simulink model "ProcessNetworkSimulation"  (R2018b)
settings: Solver=VariableStepAuto  StartTime=0.0  StopTime=2000  RelTol=1e-3  EnableMultiTasking=on
libraries: simulink x1, simeventslib x1
settings Model: Creator=tsprock3  LastModifiedBy=tas5
settings DataIOCC: LimitDataPoints=on
settings OptimizationCC: LifeSpan=inf
settings DebuggingCC: AllowSymbolicDim=off  SFUnexpectedBacktrackingDiag=warning  SFNoUnconditionalDefaultTransitionDiag=warning  SFExecutionAtInitializationDiag=none
settings ModelReferenceCC: PropagateSignalLabelsOutOfModel=off
settings SFSimCC: SimUseLocalCustomCode=off
settings RTWCC: RTWUseLocalCustomCode=off
settings CodeAppCC: StateflowObjectComments=on
settings GRTTargetCC: TargetLangStandard=C89/C90 (ANSI)
settings ConfigComp: CovMetricSettings=dw  CovHtmlReporting=on  CovSaveCumulativeToWorkspaceVar=on  CovSaveSingleToWorkspaceVar=on  CovExternalEMLEnable=off

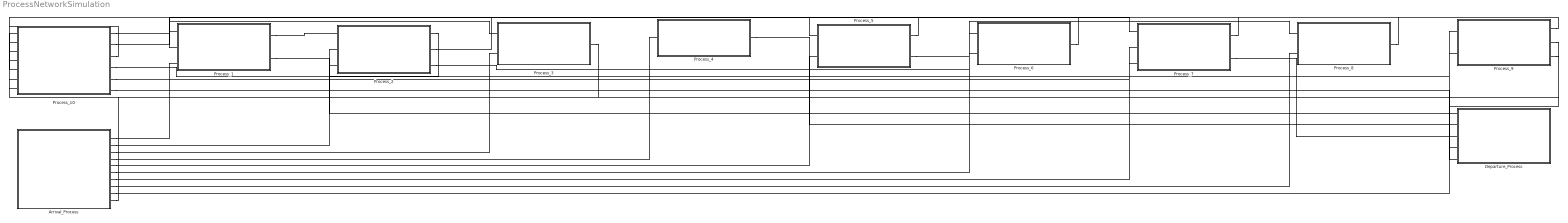
== system ProcessNetworkSimulation ==
  Arrival_Process : Subsystem
  Departure_Process : Subsystem
  Process_1 : Subsystem
  Process_10 : Subsystem
  Process_2 : Subsystem
  Process_3 : Subsystem
  Process_4 : Subsystem
  Process_5 : Subsystem
  Process_6 : Subsystem
  Process_7 : Subsystem
  Process_8 : Subsystem
  Process_9 : Subsystem
  connections:
  Process_9/RConn1 -- Process_1/LConn1
  Process_1/RConn1 -- Process_2/LConn1
  Process_2/RConn1 -- Process_2/LConn2
  Process_2/RConn2 -- Process_7/LConn1
  Process_10/RConn1 -- Process_3/LConn1
  Process_3/RConn1 -- Process_10/LConn1
  Process_10/RConn2 -- Process_5/LConn1
  Process_5/RConn1 -- Process_1/LConn2
  Process_2/RConn3 -- Process_6/LConn1
  Process_6/RConn1 -- Process_10/LConn2
  Process_10/RConn3 -- Process_10/LConn3
  Process_10/RConn4 -- Process_9/LConn1
  Process_5/RConn2 -- Process_8/LConn1
  Process_8/RConn1 -- Process_10/LConn4
  Process_7/RConn1 -- Process_10/LConn5
  Process_9/RConn2 -- Process_10/LConn6
  Process_10/RConn5 -- Process_7/LConn2
  Arrival_Process/RConn1 -- Process_1/LConn3
  Arrival_Process/RConn2 -- Process_2/LConn3
  Arrival_Process/RConn3 -- Process_3/LConn2
  Arrival_Process/RConn4 -- Process_4/LConn1
  Arrival_Process/RConn5 -- Process_5/LConn2
  Arrival_Process/RConn6 -- Process_6/LConn2
  Arrival_Process/RConn7 -- Process_7/LConn3
  Arrival_Process/RConn8 -- Process_8/LConn2
  Arrival_Process/RConn9 -- Process_9/LConn2
  Arrival_Process/RConn10 -- Process_10/LConn7
  Process_1/RConn2 -- Departure_Process/LConn1
  Process_4/RConn1 -- Departure_Process/LConn2
  Process_7/RConn2 -- Departure_Process/LConn3
  Process_9/RConn3 -- Departure_Process/LConn4
  Process_10/RConn6 -- Departure_Process/LConn5

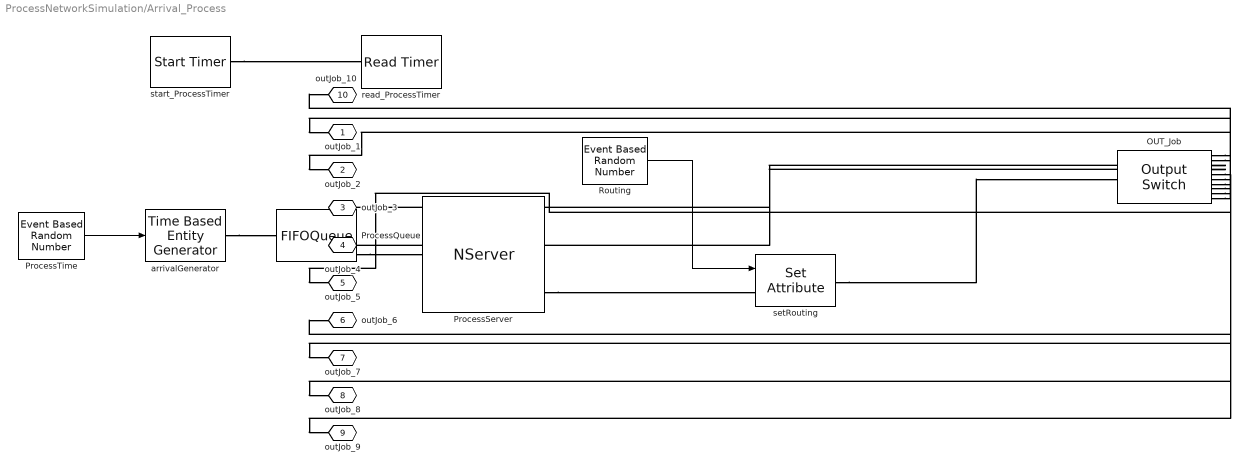
== system ProcessNetworkSimulation/Arrival_Process ==
  OUT_Job : OutputSwitch  NumberOutputPorts=10  SwitchingCriterion=From attribute  AttributeName=outputFlowNode
  ProcessQueue : FIFOQueue  Capacity=Inf  StatAverageWait=on  StatAverageQueueLength=on
      settings: OutputPortMap=o2,o3
  ProcessServer : NServer  NumberOfServers=Inf  ServiceTime=0  StatNumberDeparted=on  StatUtilization=on
      settings: OutputPortMap=o0,o5
  ProcessTime : EventBasedRandomNumber  meanExp=0.034483  minUnif=1  meanNorm=2  stdNorm=0.2  Seed=65399
  Routing : EventBasedRandomNumber  Distribution=Arbitrary discrete  valueVecDisc=[0,1,2,3,4,5,6,7,8,9,10]  probVecDisc=[0,0,0.1379,0,0,0,0,0.069,0,0.2759,0.5172]  Seed=3080
  arrivalGenerator : TimeBasedEntityGenerator  GenerateEntitiesUpon=Intergeneration time from port t
  read_ProcessTimer : ReadTimer  TimerTag=T_Arrival_Process  StatAverageTimeElapsed=on
      settings: OutputPortMap=o3
  setRouting : SetAttribute  AttributeName=outputFlowNode  AttributeFrom=Signal port  EvaluatedAttributeValue={ []}
  start_ProcessTimer : StartTimer  TimerTag=T_Arrival_Process  TimerStartedOption=Restart
  outJob_1 : PMIOPort  Side=Right
  outJob_2 : PMIOPort  Port=2  Side=Right
  outJob_3 : PMIOPort  Port=3  Side=Right
  outJob_4 : PMIOPort  Port=4  Side=Right
  outJob_5 : PMIOPort  Port=5  Side=Right
  outJob_6 : PMIOPort  Port=6  Side=Right
  outJob_7 : PMIOPort  Port=7  Side=Right
  outJob_8 : PMIOPort  Port=8  Side=Right
  outJob_9 : PMIOPort  Port=9  Side=Right
  outJob_10 : PMIOPort  Port=10  Side=Right
  wires:
  ProcessTime/1 -> arrivalGenerator/1
  Routing/1 -> setRouting/1
  connections:
  ProcessQueue/RConn1 -- ProcessServer/LConn1
  start_ProcessTimer/RConn1 -- read_ProcessTimer/LConn1
  arrivalGenerator/RConn1 -- ProcessQueue/LConn1
  ProcessServer/RConn1 -- setRouting/LConn1
  setRouting/RConn1 -- OUT_Job/LConn1
  OUT_Job/RConn1 -- outJob_1/RConn1
  OUT_Job/RConn2 -- outJob_2/RConn1
  OUT_Job/RConn3 -- outJob_3/RConn1
  OUT_Job/RConn4 -- outJob_4/RConn1
  OUT_Job/RConn5 -- outJob_5/RConn1
  OUT_Job/RConn6 -- outJob_6/RConn1
  OUT_Job/RConn7 -- outJob_7/RConn1
  OUT_Job/RConn8 -- outJob_8/RConn1
  OUT_Job/RConn9 -- outJob_9/RConn1
  OUT_Job/RConn10 -- outJob_10/RConn1

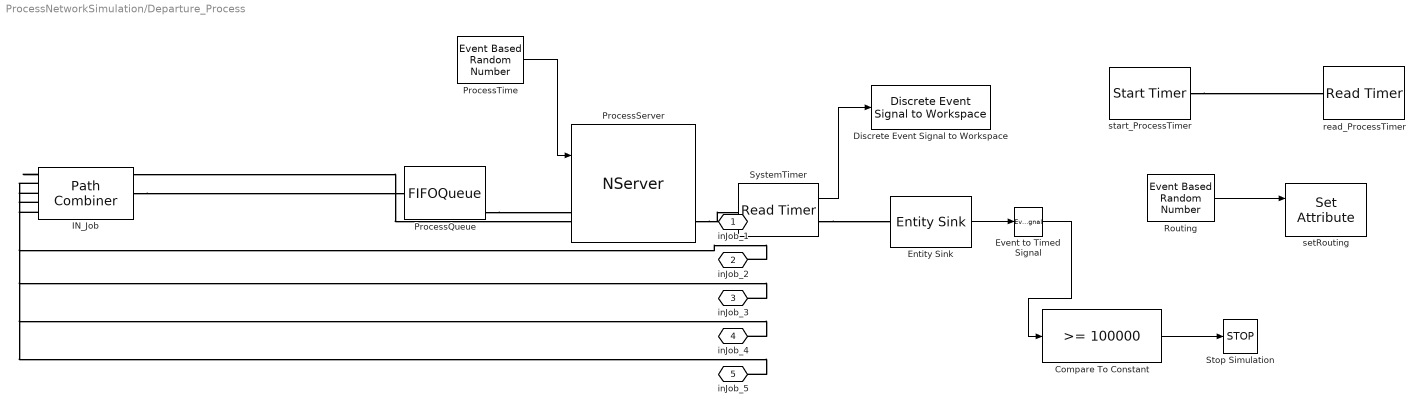
== system ProcessNetworkSimulation/Departure_Process ==
  Compare To Constant : simulink/Logic and Bit Operations/Compare To Constant  relop=>=  const=100000  OutDataTypeStr=boolean
  Discrete Event Signal to Workspace : simeventslib/SimEvents Sinks/Discrete Event Signal to Workspace  VariableName=ProcessTime  SaveFormat=Structure With Time  isMonitorOnly=off  isRecordIC=off
      settings: SourceProductName=SimEvents  SourceProductBaseCode=SE
  Entity Sink : EntitySink  StatNumberArrived=on
  Event to Timed Signal : EventToTimedSignal
  IN_Job : PathCombiner  NumberInputPorts=5
  ProcessQueue : FIFOQueue  Capacity=Inf  StatAverageWait=on  StatAverageQueueLength=on
      settings: OutputPortMap=o2,o3
  ProcessServer : NServer  NumberOfServers=Inf  ServiceTimeFrom=Signal port t  StatNumberDeparted=on  StatUtilization=on
      settings: OutputPortMap=o0,o5
  ProcessTime : EventBasedRandomNumber  Distribution=Gaussian (normal)  minUnif=1  meanNorm=0.05  stdNorm=2.2204e-16  Seed=6297
  Routing : EventBasedRandomNumber  Distribution=Arbitrary discrete  valueVecDisc=[0,1,2]  probVecDisc=[0,1,0]  Seed=9514
  Stop Simulation : Stop
  SystemTimer : ReadTimer  TimerTag=T_LHS_BU_1  TimerModeOption=Ignore  StatTimeElapsed=on
      settings: OutputPortMap=o2
  read_ProcessTimer : ReadTimer  TimerTag=T_Departure_Process  StatAverageTimeElapsed=on
      settings: OutputPortMap=o3
  setRouting : SetAttribute  AttributeName=outputFlowNode  AttributeFrom=Signal port  EvaluatedAttributeValue={ []}
  start_ProcessTimer : StartTimer  TimerTag=T_Departure_Process  TimerStartedOption=Restart
  inJob_1 : PMIOPort  Side=Left
  inJob_2 : PMIOPort  Port=2  Side=Left
  inJob_3 : PMIOPort  Port=3  Side=Left
  inJob_4 : PMIOPort  Port=4  Side=Left
  inJob_5 : PMIOPort  Port=5  Side=Left
  wires:
  SystemTimer/1 -> Discrete Event Signal to Workspace/1
  Compare To Constant/1 -> Stop Simulation/1
  Event to Timed Signal/1 -> Compare To Constant/1
  Entity Sink/1 -> Event to Timed Signal/1
  Routing/1 -> setRouting/1
  ProcessTime/1 -> ProcessServer/1
  connections:
  start_ProcessTimer/RConn1 -- read_ProcessTimer/LConn1
  SystemTimer/RConn1 -- Entity Sink/LConn1
  ProcessQueue/RConn1 -- ProcessServer/LConn1
  ProcessServer/RConn1 -- SystemTimer/LConn1
  IN_Job/RConn1 -- ProcessQueue/LConn1
  IN_Job/LConn1 -- inJob_1/RConn1
  IN_Job/LConn2 -- inJob_2/RConn1
  IN_Job/LConn3 -- inJob_3/RConn1
  IN_Job/LConn4 -- inJob_4/RConn1
  IN_Job/LConn5 -- inJob_5/RConn1

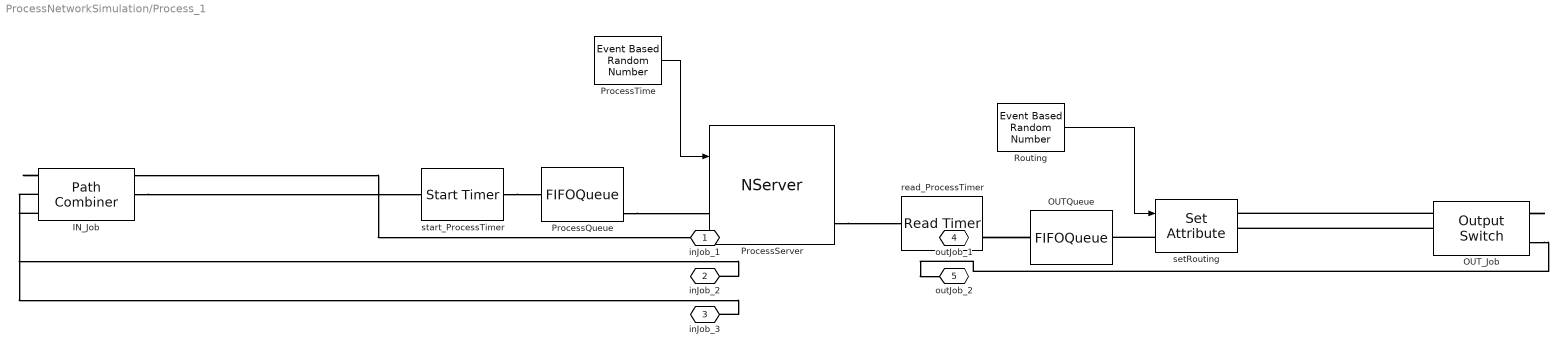
== system ProcessNetworkSimulation/Process_1 ==
  IN_Job : PathCombiner
  OUTQueue : FIFOQueue  Capacity=inf
  OUT_Job : OutputSwitch  NumberOutputPorts=2  SwitchingCriterion=From attribute  AttributeName=outputFlowNode
  ProcessQueue : FIFOQueue  Capacity=Inf  StatAverageWait=on  StatAverageQueueLength=on
      settings: OutputPortMap=o2,o3
  ProcessServer : NServer  NumberOfServers=2  ServiceTimeFrom=Signal port t  StatNumberDeparted=on  StatUtilization=on
      settings: OutputPortMap=o0,o5
  ProcessTime : EventBasedRandomNumber  meanExp=0.1  minUnif=1  meanNorm=2  stdNorm=0.2  Seed=12731
  Routing : EventBasedRandomNumber  Distribution=Arbitrary discrete  valueVecDisc=[0,1,2]  probVecDisc=[0,0.5,0.5]  Seed=15948
  read_ProcessTimer : ReadTimer  TimerTag=T_Process_1  StatAverageTimeElapsed=on
      settings: OutputPortMap=o3
  setRouting : SetAttribute  AttributeName=outputFlowNode  AttributeFrom=Signal port  EvaluatedAttributeValue={ []}
  start_ProcessTimer : StartTimer  TimerTag=T_Process_1  TimerStartedOption=Restart
  inJob_1 : PMIOPort  Side=Left
  inJob_2 : PMIOPort  Port=2  Side=Left
  inJob_3 : PMIOPort  Port=3  Side=Left
  outJob_1 : PMIOPort  Port=4  Side=Right
  outJob_2 : PMIOPort  Port=5  Side=Right
  wires:
  ProcessTime/1 -> ProcessServer/1
  Routing/1 -> setRouting/1
  connections:
  OUT_Job/LConn1 -- setRouting/RConn1
  read_ProcessTimer/RConn1 -- OUTQueue/LConn1
  ProcessQueue/RConn1 -- ProcessServer/LConn1
  start_ProcessTimer/RConn1 -- ProcessQueue/LConn1
  ProcessServer/RConn1 -- read_ProcessTimer/LConn1
  IN_Job/RConn1 -- start_ProcessTimer/LConn1
  setRouting/LConn1 -- OUTQueue/RConn1
  IN_Job/LConn1 -- inJob_1/RConn1
  IN_Job/LConn2 -- inJob_2/RConn1
  IN_Job/LConn3 -- inJob_3/RConn1
  OUT_Job/RConn1 -- outJob_1/RConn1
  OUT_Job/RConn2 -- outJob_2/RConn1

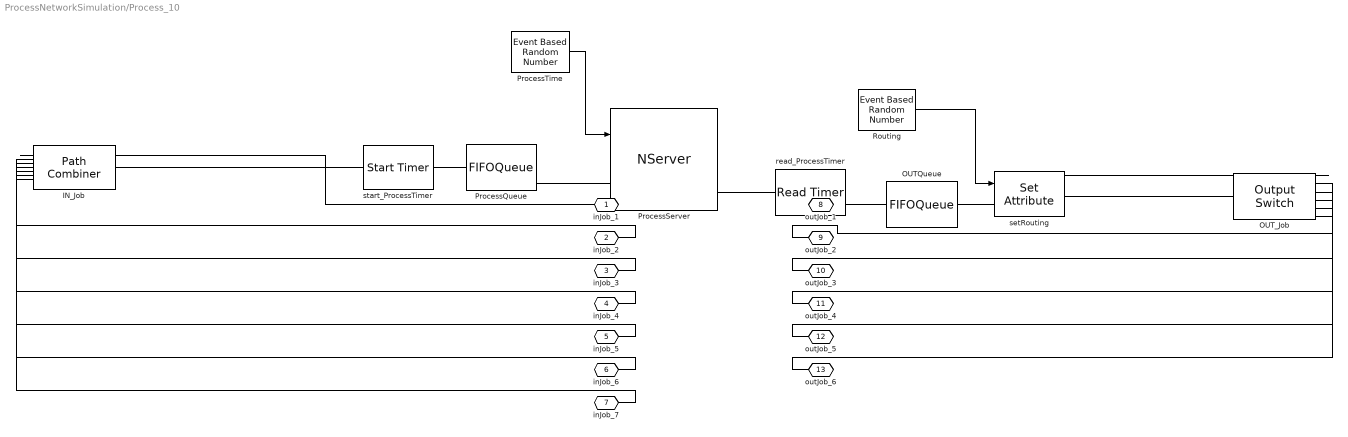
== system ProcessNetworkSimulation/Process_10 ==
  IN_Job : PathCombiner  NumberInputPorts=7
  OUTQueue : FIFOQueue  Capacity=inf
  OUT_Job : OutputSwitch  NumberOutputPorts=6  SwitchingCriterion=From attribute  AttributeName=outputFlowNode
  ProcessQueue : FIFOQueue  Capacity=Inf  StatAverageWait=on  StatAverageQueueLength=on
      settings: OutputPortMap=o2,o3
  ProcessServer : NServer  NumberOfServers=14  ServiceTimeFrom=Signal port t  StatNumberDeparted=on  StatUtilization=on
      settings: OutputPortMap=o0,o5
  ProcessTime : EventBasedRandomNumber  meanExp=0.22  minUnif=1  meanNorm=2  stdNorm=0.2  Seed=19165
  Routing : EventBasedRandomNumber  Distribution=Arbitrary discrete  valueVecDisc=[0,1,2,3,4,5,6]  probVecDisc=[0,0.2425,0.2121,0.0606,0.0606,0.2121,0.2121]  Seed=22382
  read_ProcessTimer : ReadTimer  TimerTag=T_Process_10  StatAverageTimeElapsed=on
      settings: OutputPortMap=o3
  setRouting : SetAttribute  AttributeName=outputFlowNode  AttributeFrom=Signal port  EvaluatedAttributeValue={ []}
  start_ProcessTimer : StartTimer  TimerTag=T_Process_10  TimerStartedOption=Restart
  inJob_1 : PMIOPort  Side=Left
  inJob_2 : PMIOPort  Port=2  Side=Left
  inJob_3 : PMIOPort  Port=3  Side=Left
  inJob_4 : PMIOPort  Port=4  Side=Left
  inJob_5 : PMIOPort  Port=5  Side=Left
  inJob_6 : PMIOPort  Port=6  Side=Left
  inJob_7 : PMIOPort  Port=7  Side=Left
  outJob_1 : PMIOPort  Port=8  Side=Right
  outJob_2 : PMIOPort  Port=9  Side=Right
  outJob_3 : PMIOPort  Port=10  Side=Right
  outJob_4 : PMIOPort  Port=11  Side=Right
  outJob_5 : PMIOPort  Port=12  Side=Right
  outJob_6 : PMIOPort  Port=13  Side=Right
  wires:
  ProcessTime/1 -> ProcessServer/1
  Routing/1 -> setRouting/1
  connections:
  OUT_Job/LConn1 -- setRouting/RConn1
  read_ProcessTimer/RConn1 -- OUTQueue/LConn1
  ProcessQueue/RConn1 -- ProcessServer/LConn1
  start_ProcessTimer/RConn1 -- ProcessQueue/LConn1
  ProcessServer/RConn1 -- read_ProcessTimer/LConn1
  IN_Job/RConn1 -- start_ProcessTimer/LConn1
  setRouting/LConn1 -- OUTQueue/RConn1
  IN_Job/LConn1 -- inJob_1/RConn1
  IN_Job/LConn2 -- inJob_2/RConn1
  IN_Job/LConn3 -- inJob_3/RConn1
  IN_Job/LConn4 -- inJob_4/RConn1
  IN_Job/LConn5 -- inJob_5/RConn1
  IN_Job/LConn6 -- inJob_6/RConn1
  IN_Job/LConn7 -- inJob_7/RConn1
  OUT_Job/RConn1 -- outJob_1/RConn1
  OUT_Job/RConn2 -- outJob_2/RConn1
  OUT_Job/RConn3 -- outJob_3/RConn1
  OUT_Job/RConn4 -- outJob_4/RConn1
  OUT_Job/RConn5 -- outJob_5/RConn1
  OUT_Job/RConn6 -- outJob_6/RConn1

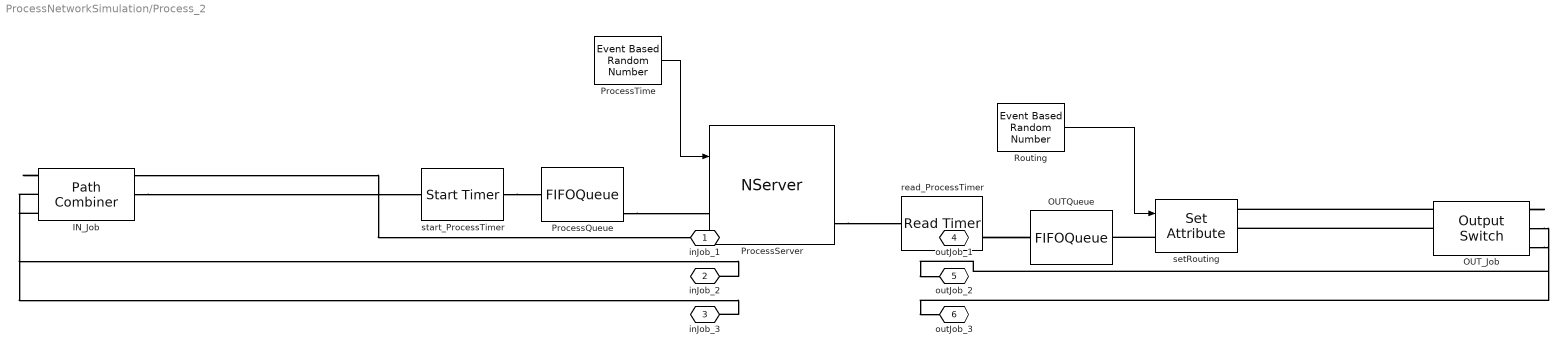
== system ProcessNetworkSimulation/Process_2 ==
  IN_Job : PathCombiner
  OUTQueue : FIFOQueue  Capacity=inf
  OUT_Job : OutputSwitch  SwitchingCriterion=From attribute  AttributeName=outputFlowNode
  ProcessQueue : FIFOQueue  Capacity=Inf  StatAverageWait=on  StatAverageQueueLength=on
      settings: OutputPortMap=o2,o3
  ProcessServer : NServer  ServiceTimeFrom=Signal port t  StatNumberDeparted=on  StatUtilization=on
      settings: OutputPortMap=o0,o5
  ProcessTime : EventBasedRandomNumber  meanExp=0.2  minUnif=1  meanNorm=2  stdNorm=0.2  Seed=25599
  Routing : EventBasedRandomNumber  Distribution=Arbitrary discrete  valueVecDisc=[0,1,2,3,4]  probVecDisc=[0,0.4,0.2,0.4,0]  Seed=28816
  read_ProcessTimer : ReadTimer  TimerTag=T_Process_2  StatAverageTimeElapsed=on
      settings: OutputPortMap=o3
  setRouting : SetAttribute  AttributeName=outputFlowNode  AttributeFrom=Signal port  EvaluatedAttributeValue={ []}
  start_ProcessTimer : StartTimer  TimerTag=T_Process_2  TimerStartedOption=Restart
  inJob_1 : PMIOPort  Side=Left
  inJob_2 : PMIOPort  Port=2  Side=Left
  inJob_3 : PMIOPort  Port=3  Side=Left
  outJob_1 : PMIOPort  Port=4  Side=Right
  outJob_2 : PMIOPort  Port=5  Side=Right
  outJob_3 : PMIOPort  Port=6  Side=Right
  wires:
  ProcessTime/1 -> ProcessServer/1
  Routing/1 -> setRouting/1
  connections:
  OUT_Job/LConn1 -- setRouting/RConn1
  read_ProcessTimer/RConn1 -- OUTQueue/LConn1
  ProcessQueue/RConn1 -- ProcessServer/LConn1
  start_ProcessTimer/RConn1 -- ProcessQueue/LConn1
  ProcessServer/RConn1 -- read_ProcessTimer/LConn1
  IN_Job/RConn1 -- start_ProcessTimer/LConn1
  setRouting/LConn1 -- OUTQueue/RConn1
  IN_Job/LConn1 -- inJob_1/RConn1
  IN_Job/LConn2 -- inJob_2/RConn1
  IN_Job/LConn3 -- inJob_3/RConn1
  OUT_Job/RConn1 -- outJob_1/RConn1
  OUT_Job/RConn2 -- outJob_2/RConn1
  OUT_Job/RConn3 -- outJob_3/RConn1

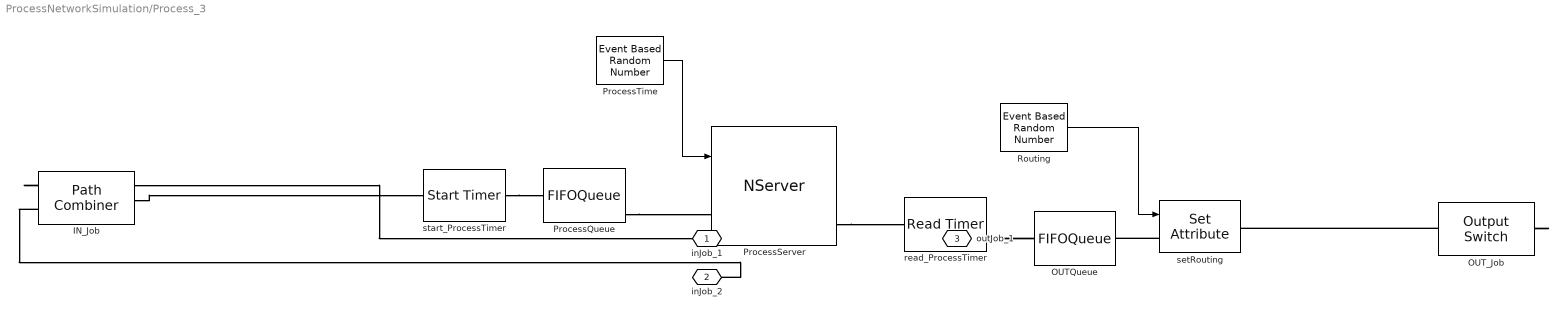
== system ProcessNetworkSimulation/Process_3 ==
  IN_Job : PathCombiner  NumberInputPorts=2
  OUTQueue : FIFOQueue  Capacity=inf
  OUT_Job : OutputSwitch  NumberOutputPorts=1  SwitchingCriterion=From attribute  AttributeName=outputFlowNode
  ProcessQueue : FIFOQueue  Capacity=Inf  StatAverageWait=on  StatAverageQueueLength=on
      settings: OutputPortMap=o2,o3
  ProcessServer : NServer  NumberOfServers=4  ServiceTimeFrom=Signal port t  StatNumberDeparted=on  StatUtilization=on
      settings: OutputPortMap=o0,o5
  ProcessTime : EventBasedRandomNumber  meanExp=0.22  minUnif=1  meanNorm=2  stdNorm=0.2  Seed=32033
  Routing : EventBasedRandomNumber  Distribution=Arbitrary discrete  valueVecDisc=[0,1,2]  probVecDisc=[0,1,0]  Seed=35250
  read_ProcessTimer : ReadTimer  TimerTag=T_Process_3  StatAverageTimeElapsed=on
      settings: OutputPortMap=o3
  setRouting : SetAttribute  AttributeName=outputFlowNode  AttributeFrom=Signal port  EvaluatedAttributeValue={ []}
  start_ProcessTimer : StartTimer  TimerTag=T_Process_3  TimerStartedOption=Restart
  inJob_1 : PMIOPort  Side=Left
  inJob_2 : PMIOPort  Port=2  Side=Left
  outJob_1 : PMIOPort  Port=3  Side=Right
  wires:
  ProcessTime/1 -> ProcessServer/1
  Routing/1 -> setRouting/1
  connections:
  OUT_Job/LConn1 -- setRouting/RConn1
  read_ProcessTimer/RConn1 -- OUTQueue/LConn1
  ProcessQueue/RConn1 -- ProcessServer/LConn1
  start_ProcessTimer/RConn1 -- ProcessQueue/LConn1
  ProcessServer/RConn1 -- read_ProcessTimer/LConn1
  IN_Job/RConn1 -- start_ProcessTimer/LConn1
  setRouting/LConn1 -- OUTQueue/RConn1
  IN_Job/LConn1 -- inJob_1/RConn1
  IN_Job/LConn2 -- inJob_2/RConn1
  OUT_Job/RConn1 -- outJob_1/RConn1

== system ProcessNetworkSimulation/Process_4 ==
  IN_Job : PathCombiner  NumberInputPorts=1
  OUTQueue : FIFOQueue  Capacity=inf
  OUT_Job : OutputSwitch  NumberOutputPorts=1  SwitchingCriterion=From attribute  AttributeName=outputFlowNode
  ProcessQueue : FIFOQueue  Capacity=Inf  StatAverageWait=on  StatAverageQueueLength=on
      settings: OutputPortMap=o2,o3
  ProcessServer : NServer  NumberOfServers=1  ServiceTimeFrom=Signal port t  StatNumberDeparted=on  StatUtilization=on
      settings: OutputPortMap=o0,o5
  ProcessTime : EventBasedRandomNumber  meanExp=0.12  minUnif=1  meanNorm=2  stdNorm=0.2  Seed=38467
  Routing : EventBasedRandomNumber  Distribution=Arbitrary discrete  valueVecDisc=[0,1]  probVecDisc=[0,1]  Seed=41684
  read_ProcessTimer : ReadTimer  TimerTag=T_Process_4  StatAverageTimeElapsed=on
      settings: OutputPortMap=o3
  setRouting : SetAttribute  AttributeName=outputFlowNode  AttributeFrom=Signal port  EvaluatedAttributeValue={ []}
  start_ProcessTimer : StartTimer  TimerTag=T_Process_4  TimerStartedOption=Restart
  inJob_1 : PMIOPort  Side=Left
  outJob_1 : PMIOPort  Port=2  Side=Right
  wires:
  ProcessTime/1 -> ProcessServer/1
  Routing/1 -> setRouting/1
  connections:
  OUT_Job/LConn1 -- setRouting/RConn1
  read_ProcessTimer/RConn1 -- OUTQueue/LConn1
  ProcessQueue/RConn1 -- ProcessServer/LConn1
  start_ProcessTimer/RConn1 -- ProcessQueue/LConn1
  ProcessServer/RConn1 -- read_ProcessTimer/LConn1
  IN_Job/RConn1 -- start_ProcessTimer/LConn1
  setRouting/LConn1 -- OUTQueue/RConn1
  IN_Job/LConn1 -- inJob_1/RConn1
  OUT_Job/RConn1 -- outJob_1/RConn1

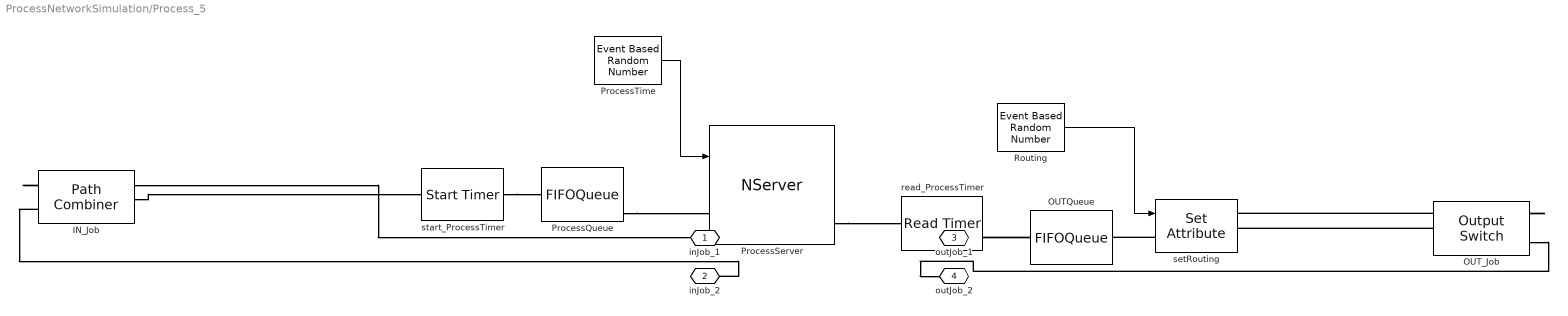
== system ProcessNetworkSimulation/Process_5 ==
  IN_Job : PathCombiner  NumberInputPorts=2
  OUTQueue : FIFOQueue  Capacity=inf
  OUT_Job : OutputSwitch  NumberOutputPorts=2  SwitchingCriterion=From attribute  AttributeName=outputFlowNode
  ProcessQueue : FIFOQueue  Capacity=Inf  StatAverageWait=on  StatAverageQueueLength=on
      settings: OutputPortMap=o2,o3
  ProcessServer : NServer  NumberOfServers=1  ServiceTimeFrom=Signal port t  StatNumberDeparted=on  StatUtilization=on
      settings: OutputPortMap=o0,o5
  ProcessTime : EventBasedRandomNumber  meanExp=0.06  minUnif=1  meanNorm=2  stdNorm=0.2  Seed=44901
  Routing : EventBasedRandomNumber  Distribution=Arbitrary discrete  valueVecDisc=[0,1,2,3]  probVecDisc=[0,0.5333,0.4667,0]  Seed=48118
  read_ProcessTimer : ReadTimer  TimerTag=T_Process_5  StatAverageTimeElapsed=on
      settings: OutputPortMap=o3
  setRouting : SetAttribute  AttributeName=outputFlowNode  AttributeFrom=Signal port  EvaluatedAttributeValue={ []}
  start_ProcessTimer : StartTimer  TimerTag=T_Process_5  TimerStartedOption=Restart
  inJob_1 : PMIOPort  Side=Left
  inJob_2 : PMIOPort  Port=2  Side=Left
  outJob_1 : PMIOPort  Port=3  Side=Right
  outJob_2 : PMIOPort  Port=4  Side=Right
  wires:
  ProcessTime/1 -> ProcessServer/1
  Routing/1 -> setRouting/1
  connections:
  OUT_Job/LConn1 -- setRouting/RConn1
  read_ProcessTimer/RConn1 -- OUTQueue/LConn1
  ProcessQueue/RConn1 -- ProcessServer/LConn1
  start_ProcessTimer/RConn1 -- ProcessQueue/LConn1
  ProcessServer/RConn1 -- read_ProcessTimer/LConn1
  IN_Job/RConn1 -- start_ProcessTimer/LConn1
  setRouting/LConn1 -- OUTQueue/RConn1
  IN_Job/LConn1 -- inJob_1/RConn1
  IN_Job/LConn2 -- inJob_2/RConn1
  OUT_Job/RConn1 -- outJob_1/RConn1
  OUT_Job/RConn2 -- outJob_2/RConn1

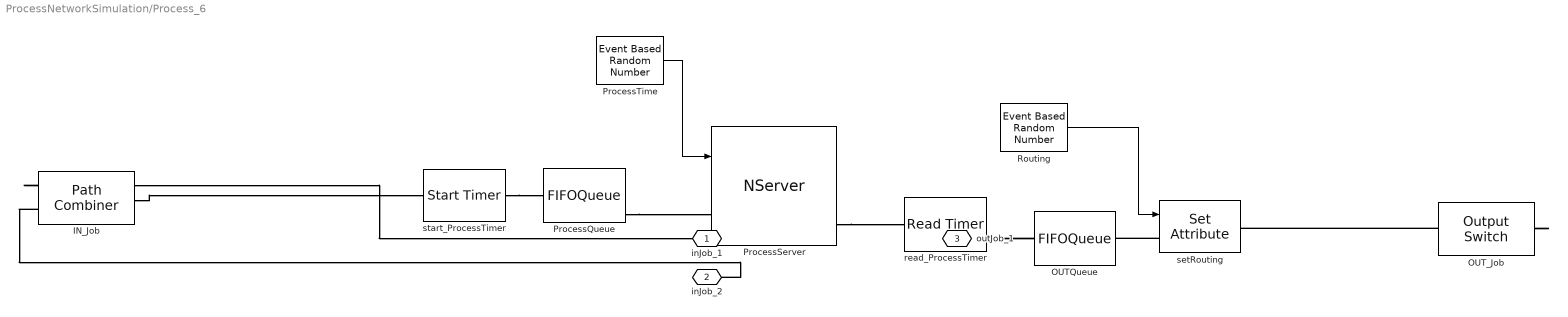
== system ProcessNetworkSimulation/Process_6 ==
  IN_Job : PathCombiner  NumberInputPorts=2
  OUTQueue : FIFOQueue  Capacity=inf
  OUT_Job : OutputSwitch  NumberOutputPorts=1  SwitchingCriterion=From attribute  AttributeName=outputFlowNode
  ProcessQueue : FIFOQueue  Capacity=Inf  StatAverageWait=on  StatAverageQueueLength=on
      settings: OutputPortMap=o2,o3
  ProcessServer : NServer  NumberOfServers=1  ServiceTimeFrom=Signal port t  StatNumberDeparted=on  StatUtilization=on
      settings: OutputPortMap=o0,o5
  ProcessTime : EventBasedRandomNumber  meanExp=0.08  minUnif=1  meanNorm=2  stdNorm=0.2  Seed=51335
  Routing : EventBasedRandomNumber  Distribution=Arbitrary discrete  valueVecDisc=[0,1,2]  probVecDisc=[0,1,0]  Seed=54552
  read_ProcessTimer : ReadTimer  TimerTag=T_Process_6  StatAverageTimeElapsed=on
      settings: OutputPortMap=o3
  setRouting : SetAttribute  AttributeName=outputFlowNode  AttributeFrom=Signal port  EvaluatedAttributeValue={ []}
  start_ProcessTimer : StartTimer  TimerTag=T_Process_6  TimerStartedOption=Restart
  inJob_1 : PMIOPort  Side=Left
  inJob_2 : PMIOPort  Port=2  Side=Left
  outJob_1 : PMIOPort  Port=3  Side=Right
  wires:
  ProcessTime/1 -> ProcessServer/1
  Routing/1 -> setRouting/1
  connections:
  OUT_Job/LConn1 -- setRouting/RConn1
  read_ProcessTimer/RConn1 -- OUTQueue/LConn1
  ProcessQueue/RConn1 -- ProcessServer/LConn1
  start_ProcessTimer/RConn1 -- ProcessQueue/LConn1
  ProcessServer/RConn1 -- read_ProcessTimer/LConn1
  IN_Job/RConn1 -- start_ProcessTimer/LConn1
  setRouting/LConn1 -- OUTQueue/RConn1
  IN_Job/LConn1 -- inJob_1/RConn1
  IN_Job/LConn2 -- inJob_2/RConn1
  OUT_Job/RConn1 -- outJob_1/RConn1

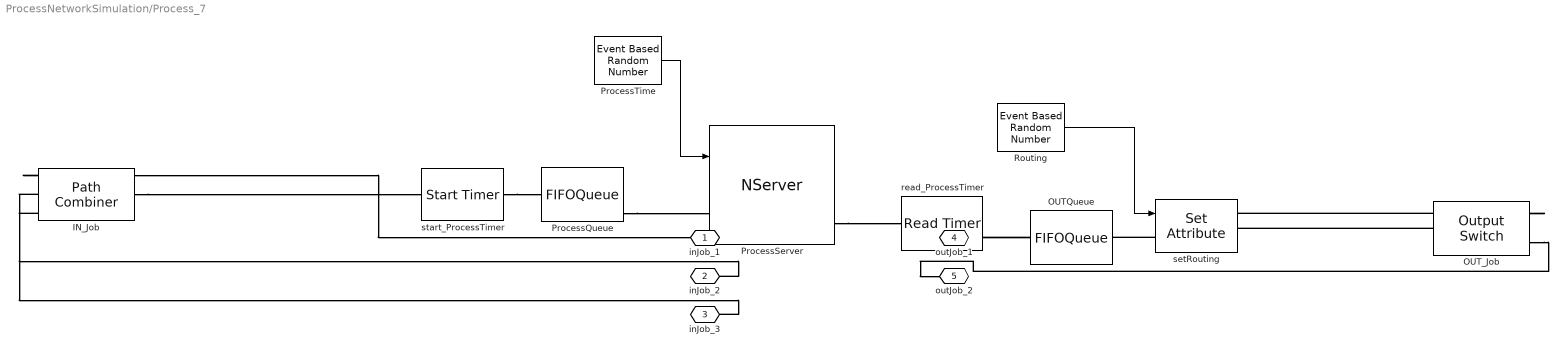
== system ProcessNetworkSimulation/Process_7 ==
  IN_Job : PathCombiner
  OUTQueue : FIFOQueue  Capacity=inf
  OUT_Job : OutputSwitch  NumberOutputPorts=2  SwitchingCriterion=From attribute  AttributeName=outputFlowNode
  ProcessQueue : FIFOQueue  Capacity=Inf  StatAverageWait=on  StatAverageQueueLength=on
      settings: OutputPortMap=o2,o3
  ProcessServer : NServer  NumberOfServers=3  ServiceTimeFrom=Signal port t  StatNumberDeparted=on  StatUtilization=on
      settings: OutputPortMap=o0,o5
  ProcessTime : EventBasedRandomNumber  meanExp=0.14  minUnif=1  meanNorm=2  stdNorm=0.2  Seed=57769
  Routing : EventBasedRandomNumber  Distribution=Arbitrary discrete  valueVecDisc=[0,1,2]  probVecDisc=[0,0.1667,0.8333]  Seed=60986
  read_ProcessTimer : ReadTimer  TimerTag=T_Process_7  StatAverageTimeElapsed=on
      settings: OutputPortMap=o3
  setRouting : SetAttribute  AttributeName=outputFlowNode  AttributeFrom=Signal port  EvaluatedAttributeValue={ []}
  start_ProcessTimer : StartTimer  TimerTag=T_Process_7  TimerStartedOption=Restart
  inJob_1 : PMIOPort  Side=Left
  inJob_2 : PMIOPort  Port=2  Side=Left
  inJob_3 : PMIOPort  Port=3  Side=Left
  outJob_1 : PMIOPort  Port=4  Side=Right
  outJob_2 : PMIOPort  Port=5  Side=Right
  wires:
  ProcessTime/1 -> ProcessServer/1
  Routing/1 -> setRouting/1
  connections:
  OUT_Job/LConn1 -- setRouting/RConn1
  read_ProcessTimer/RConn1 -- OUTQueue/LConn1
  ProcessQueue/RConn1 -- ProcessServer/LConn1
  start_ProcessTimer/RConn1 -- ProcessQueue/LConn1
  ProcessServer/RConn1 -- read_ProcessTimer/LConn1
  IN_Job/RConn1 -- start_ProcessTimer/LConn1
  setRouting/LConn1 -- OUTQueue/RConn1
  IN_Job/LConn1 -- inJob_1/RConn1
  IN_Job/LConn2 -- inJob_2/RConn1
  IN_Job/LConn3 -- inJob_3/RConn1
  OUT_Job/RConn1 -- outJob_1/RConn1
  OUT_Job/RConn2 -- outJob_2/RConn1

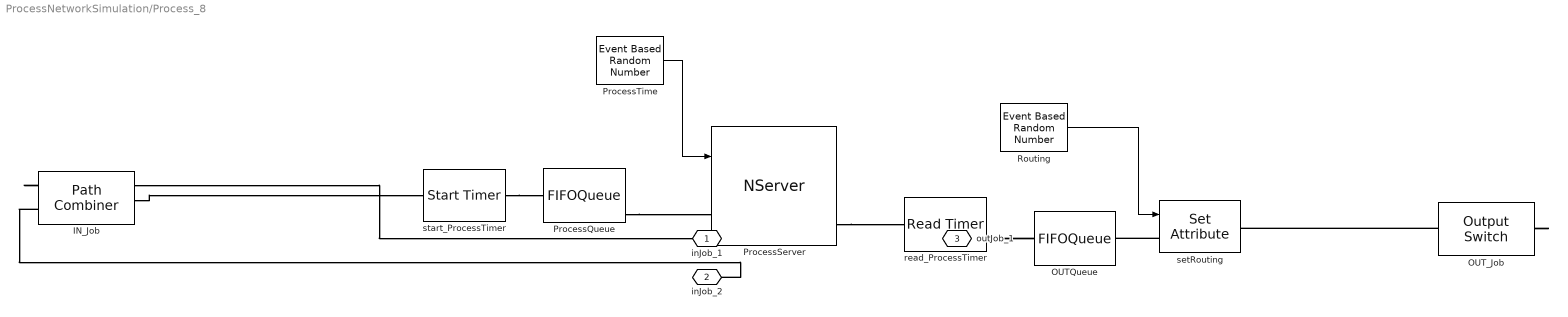
== system ProcessNetworkSimulation/Process_8 ==
  IN_Job : PathCombiner  NumberInputPorts=2
  OUTQueue : FIFOQueue  Capacity=inf
  OUT_Job : OutputSwitch  NumberOutputPorts=1  SwitchingCriterion=From attribute  AttributeName=outputFlowNode
  ProcessQueue : FIFOQueue  Capacity=Inf  StatAverageWait=on  StatAverageQueueLength=on
      settings: OutputPortMap=o2,o3
  ProcessServer : NServer  NumberOfServers=1  ServiceTimeFrom=Signal port t  StatNumberDeparted=on  StatUtilization=on
      settings: OutputPortMap=o0,o5
  ProcessTime : EventBasedRandomNumber  meanExp=0.07  minUnif=1  meanNorm=2  stdNorm=0.2  Seed=64203
  Routing : EventBasedRandomNumber  Distribution=Arbitrary discrete  valueVecDisc=[0,1,2]  probVecDisc=[0,1,0]  Seed=1884
  read_ProcessTimer : ReadTimer  TimerTag=T_Process_8  StatAverageTimeElapsed=on
      settings: OutputPortMap=o3
  setRouting : SetAttribute  AttributeName=outputFlowNode  AttributeFrom=Signal port  EvaluatedAttributeValue={ []}
  start_ProcessTimer : StartTimer  TimerTag=T_Process_8  TimerStartedOption=Restart
  inJob_1 : PMIOPort  Side=Left
  inJob_2 : PMIOPort  Port=2  Side=Left
  outJob_1 : PMIOPort  Port=3  Side=Right
  wires:
  ProcessTime/1 -> ProcessServer/1
  Routing/1 -> setRouting/1
  connections:
  OUT_Job/LConn1 -- setRouting/RConn1
  read_ProcessTimer/RConn1 -- OUTQueue/LConn1
  ProcessQueue/RConn1 -- ProcessServer/LConn1
  start_ProcessTimer/RConn1 -- ProcessQueue/LConn1
  ProcessServer/RConn1 -- read_ProcessTimer/LConn1
  IN_Job/RConn1 -- start_ProcessTimer/LConn1
  setRouting/LConn1 -- OUTQueue/RConn1
  IN_Job/LConn1 -- inJob_1/RConn1
  IN_Job/LConn2 -- inJob_2/RConn1
  OUT_Job/RConn1 -- outJob_1/RConn1

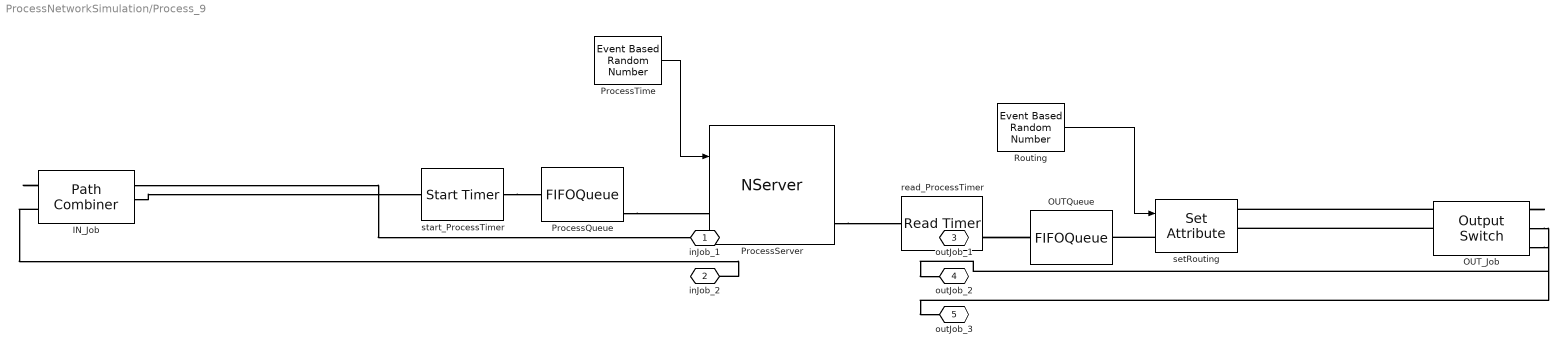
== system ProcessNetworkSimulation/Process_9 ==
  IN_Job : PathCombiner  NumberInputPorts=2
  OUTQueue : FIFOQueue  Capacity=inf
  OUT_Job : OutputSwitch  SwitchingCriterion=From attribute  AttributeName=outputFlowNode
  ProcessQueue : FIFOQueue  Capacity=Inf  StatAverageWait=on  StatAverageQueueLength=on
      settings: OutputPortMap=o2,o3
  ProcessServer : NServer  NumberOfServers=2  ServiceTimeFrom=Signal port t  StatNumberDeparted=on  StatUtilization=on
      settings: OutputPortMap=o0,o5
  ProcessTime : EventBasedRandomNumber  meanExp=0.14  minUnif=1  meanNorm=2  stdNorm=0.2  Seed=5101
  Routing : EventBasedRandomNumber  Distribution=Arbitrary discrete  valueVecDisc=[0,1,2,3]  probVecDisc=[0,0.5714,0.1429,0.2857]  Seed=8318
  read_ProcessTimer : ReadTimer  TimerTag=T_Process_9  StatAverageTimeElapsed=on
      settings: OutputPortMap=o3
  setRouting : SetAttribute  AttributeName=outputFlowNode  AttributeFrom=Signal port  EvaluatedAttributeValue={ []}
  start_ProcessTimer : StartTimer  TimerTag=T_Process_9  TimerStartedOption=Restart
  inJob_1 : PMIOPort  Side=Left
  inJob_2 : PMIOPort  Port=2  Side=Left
  outJob_1 : PMIOPort  Port=3  Side=Right
  outJob_2 : PMIOPort  Port=4  Side=Right
  outJob_3 : PMIOPort  Port=5  Side=Right
  wires:
  ProcessTime/1 -> ProcessServer/1
  Routing/1 -> setRouting/1
  connections:
  OUT_Job/LConn1 -- setRouting/RConn1
  read_ProcessTimer/RConn1 -- OUTQueue/LConn1
  ProcessQueue/RConn1 -- ProcessServer/LConn1
  start_ProcessTimer/RConn1 -- ProcessQueue/LConn1
  ProcessServer/RConn1 -- read_ProcessTimer/LConn1
  IN_Job/RConn1 -- start_ProcessTimer/LConn1
  setRouting/LConn1 -- OUTQueue/RConn1
  IN_Job/LConn1 -- inJob_1/RConn1
  IN_Job/LConn2 -- inJob_2/RConn1
  OUT_Job/RConn1 -- outJob_1/RConn1
  OUT_Job/RConn2 -- outJob_2/RConn1
  OUT_Job/RConn3 -- outJob_3/RConn1
